simulink model "threebus"  (R2024a)
settings: Solver=VariableStepAuto  StartTime=0.0  StopTime=10.0  RelTol=1e-3
libraries: spsThreePhaseVIMeasurementLib x6, spsThreePhaseSeriesRLCBranchLib x3, spsLoadFlowBusLib x3, spsThreePhaseParallelRLCLoadLib x2, spsThreePhaseBreakerLib x1, spsThreePhaseSourceLib x1, sps_lib x1
settings Model: Creator=Vaibhav Chaudhary  LastModifiedBy=Vaibhav Chaudhary

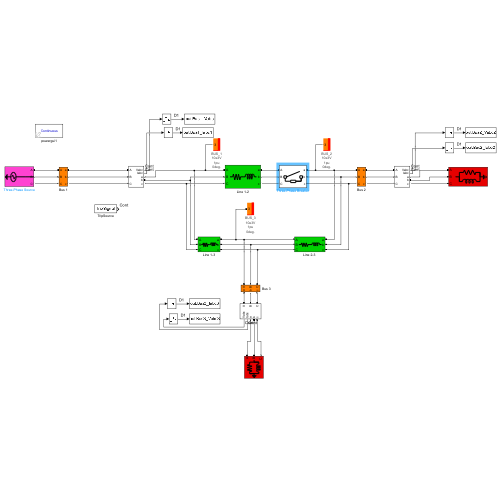
[thumbnail: Simulink's stored preview of the top-level diagram]
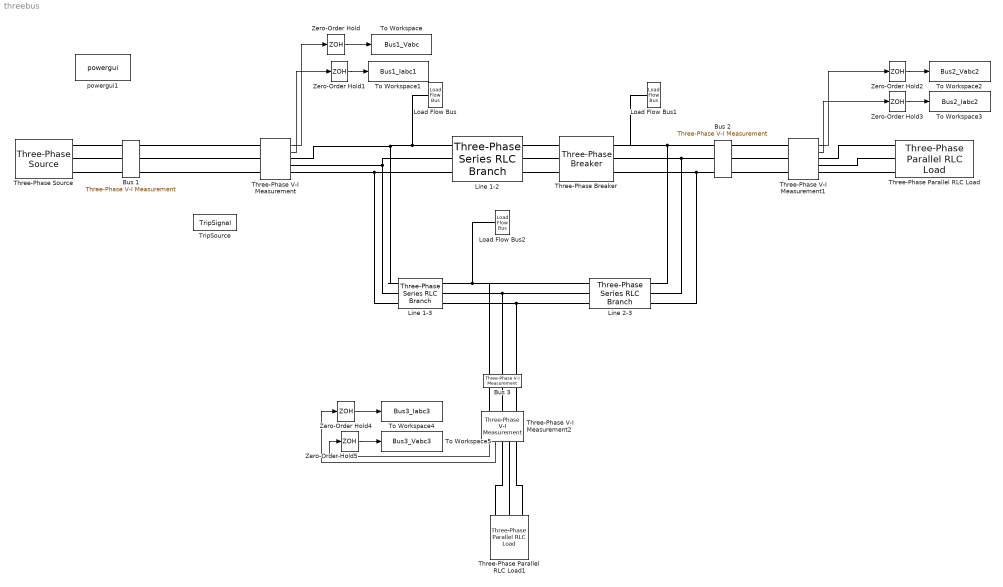
== system threebus ==
  Bus 1 : spsThreePhaseVIMeasurementLib/Three-Phase V-I Measurement  VoltageMeasurement=no  SetLabelV=off  LabelV=Vabc  Vpu=off  VpuLL=off  CurrentMeasurement=no  SetLabelI=off  LabelI=Iabc  Ipu=off  Pbase=100e6  Vbase=500e3  OutputType=Complex  PhasorSimulation=off  PSBequivalent=0
  Bus 2 : spsThreePhaseVIMeasurementLib/Three-Phase V-I Measurement  VoltageMeasurement=no  SetLabelV=off  LabelV=Vabc  Vpu=off  VpuLL=off  CurrentMeasurement=no  SetLabelI=off  LabelI=Iabc  Ipu=off  Pbase=100e6  Vbase=500e3  OutputType=Complex  PhasorSimulation=off  PSBequivalent=0
  Bus 3 : spsThreePhaseVIMeasurementLib/Three-Phase V-I Measurement  VoltageMeasurement=no  SetLabelV=off  LabelV=Vabc  Vpu=off  VpuLL=off  CurrentMeasurement=no  SetLabelI=off  LabelI=Iabc  Ipu=off  Pbase=100e6  Vbase=500e3  OutputType=Complex  PhasorSimulation=off  PSBequivalent=0
  Line 1-2 : spsThreePhaseSeriesRLCBranchLib/Three-Phase Series RLC Branch  LConnTagsString=A|B|C  RConnTagsString=A|B|C  BranchType=RL  Resistance=0.02  Inductance=106.1e-6  Capacitance=1e-6  Measurements=None
  Line 1-3 : spsThreePhaseSeriesRLCBranchLib/Three-Phase Series RLC Branch  LConnTagsString=A|B|C  RConnTagsString=A|B|C  BranchType=RL  Resistance=0.01  Inductance=79.577e-6  Capacitance=1e-6  Measurements=None
  "Line 2-3 " : spsThreePhaseSeriesRLCBranchLib/Three-Phase Series RLC Branch  LConnTagsString=A|B|C  RConnTagsString=A|B|C  BranchType=RL  Resistance=0.01  Inductance=66.31e-6  Capacitance=1e-6  Measurements=None
  Load Flow Bus : spsLoadFlowBusLib/Load Flow Bus  LConnTagsString=a  Phases=single  Connectors=on one side  ID=BUS_1  Vbase=10e3  Vref=1.05  Vangle=0  VLF=1  VLFb=1  VLFc=1  angleLF=0  angleLFb=0  angleLFc=0
  Load Flow Bus1 : spsLoadFlowBusLib/Load Flow Bus  LConnTagsString=a  Phases=single  Connectors=on one side  ID=BUS_2  Vbase=10e3  Vref=1.05  Vangle=0  VLF=1  VLFb=1  VLFc=1  angleLF=0  angleLFb=0  angleLFc=0
  Load Flow Bus2 : spsLoadFlowBusLib/Load Flow Bus  LConnTagsString=a  Phases=single  Connectors=on one side  ID=BUS_3  Vbase=10e3  Vref=1.05  Vangle=0  VLF=1  VLFb=1  VLFc=1  angleLF=0  angleLFb=0  angleLFc=0
  Three-Phase Parallel RLC Load : spsThreePhaseParallelRLCLoadLib/Three-Phase Parallel RLC Load  LConnTagsString=A|B|C  Configuration=Y (grounded)  NominalVoltage=1000  Vabc=[1e3 1e3 1e3]  Vabcp=[1e3 1e3 1e3]  NominalFrequency=60  UnbalancedPower=off  ActivePower=256.6e6  InductivePower=110.2e6  CapacitivePower=0  Pabc=[10e3 9e3 11e3]  QLabc=[100 90 110]  QCabc=[100 90 110]  Pabcp=[10e3 9e3 11e3]  QLabcp=[100 90 110]  QCabcp=[100 90 110]  Measurements=None  LoadType=constant PQ
  Three-Phase Parallel RLC Load1 : spsThreePhaseParallelRLCLoadLib/Three-Phase Parallel RLC Load  LConnTagsString=A|B|C  Configuration=Y (grounded)  NominalVoltage=1000  Vabc=[1e3 1e3 1e3]  Vabcp=[1e3 1e3 1e3]  NominalFrequency=60  UnbalancedPower=off  ActivePower=138.6e6  InductivePower=45.2e6  CapacitivePower=0  Pabc=[10e3 9e3 11e3]  QLabc=[100 90 110]  QCabc=[100 90 110]  Pabcp=[10e3 9e3 11e3]  QLabcp=[100 90 110]  QCabcp=[100 90 110]  Measurements=None  LoadType=constant PQ
  Three-Phase V-I Measurement : spsThreePhaseVIMeasurementLib/Three-Phase V-I Measurement  VoltageMeasurement=phase-to-ground  SetLabelV=off  LabelV=Vabc  Vpu=off  VpuLL=off  CurrentMeasurement=yes  SetLabelI=off  LabelI=Iabc  Ipu=off  Pbase=100e6  Vbase=500e3  OutputType=Complex  PhasorSimulation=off  PSBequivalent=0
  Three-Phase V-I Measurement1 : spsThreePhaseVIMeasurementLib/Three-Phase V-I Measurement  VoltageMeasurement=phase-to-ground  SetLabelV=off  LabelV=Vabc  Vpu=off  VpuLL=off  CurrentMeasurement=yes  SetLabelI=off  LabelI=Iabc  Ipu=off  Pbase=100e6  Vbase=500e3  OutputType=Complex  PhasorSimulation=off  PSBequivalent=0
  Three-Phase V-I Measurement2 : spsThreePhaseVIMeasurementLib/Three-Phase V-I Measurement  VoltageMeasurement=phase-to-ground  SetLabelV=off  LabelV=Vabc  Vpu=off  VpuLL=off  CurrentMeasurement=yes  SetLabelI=off  LabelI=Iabc  Ipu=off  Pbase=100e6  Vbase=500e3  OutputType=Complex  PhasorSimulation=off  PSBequivalent=0
  Three-Phase Breaker : spsThreePhaseBreakerLib/Three-Phase Breaker  InitialState=open  SwitchA=on  SwitchB=on  SwitchC=on  SwitchTimes="[1/60  5/60]"  External=off  BreakerResistance=0.01  SnubberResistance=1e6  SnubberCapacitance=inf  Measurements=None
  Three-Phase Source : spsThreePhaseSourceLib/Three-Phase Source  InternalConnection=Yg  VoltagePhases=off  Voltage=25e3  PhaseAngle=0  Voltage_phases=[25e3 25e3 25e3]/sqrt(3)  PhaseAngles_phases=[0 -120 +120]  Frequency=60  NonIdealSource=on  SpecifyImpedance=off  Resistance=0  Inductance=0  ShortCircuitLevel=100e6  BaseVoltage=25e3  XRratio=7  BusType=swing  Pref=10e3  Qref=0  Prefabc=[10e3, 10e3, 10e3]  Qrefabc=[0, 0, 0]  Qmin=-inf  Qmax=inf
  To Workspace : ToWorkspace  VariableName=Bus1_Vabc  SampleTime=-1
  To Workspace1 : ToWorkspace  VariableName=Bus1_Iabc1  SampleTime=-1
  To Workspace2 : ToWorkspace  VariableName=Bus2_Vabc2  SampleTime=-1
  To Workspace3 : ToWorkspace  VariableName=Bus2_Iabc2  SampleTime=-1
  To Workspace4 : ToWorkspace  VariableName=Bus3_Iabc3  SampleTime=-1
  To Workspace5 : ToWorkspace  VariableName=Bus3_Vabc3  SampleTime=-1
  TripSource : FromWorkspace  VariableName=TripSignal
  Zero-Order Hold{,1..5} (6 alike) : ZeroOrderHold  SampleTime=0.1
  powergui1 : sps_lib/powergui  Priority=1  SimulationMode=Continuous  SampleTime=50e-6  frequency=60  Iterations=50  frequencyindice=60  Pbase=100e6  ErrMax=1e-4  UnitsV=kV  UnitsW=MW  buscounter=0  FunctionMessages=off  echomessages=off  EnableUseOfTLC=off  CurrentSourceSwitches=off  DisableSnubberDevices=off  DisableRonSwitches=off  DisableVfSwitches=off  DisplayEquations=off  AutomaticDiscreteSolvers=off  SolverType=Tustin/Backward Euler (TBE)  Interpol=off  ExternalGateDelay=off  methode=off  Ts=100  x0status=blocks  SPID=on  SwTol=0  HookPort=off  NonlinearTolerance=1e-4  nMaxIteration=100  ContinueOnMaxIteration=off  RestoreLinks=warning  ResistiveCurrentMeasurement=off  Frange=[0:2:500]  Ylog=off  Xlog=on  ShowGrid=off  save=off  variable=ZData  structure=0  ZoomFFT=off  StartTime=0.0  cycles=1  DisplayStyle=1  fundamental=60  FreqAxis=off  MaxFrequency=1000  frequencyindicesteady=1  RmsSteady=1  display=off
  wires:
  Zero-Order Hold/1 -> To Workspace/1
  Three-Phase V-I Measurement/1 -> Zero-Order Hold/1
  Zero-Order Hold1/1 -> To Workspace1/1
  Three-Phase V-I Measurement/2 -> Zero-Order Hold1/1
  Zero-Order Hold2/1 -> To Workspace2/1
  Three-Phase V-I Measurement1/1 -> Zero-Order Hold2/1
  Zero-Order Hold3/1 -> To Workspace3/1
  Three-Phase V-I Measurement1/2 -> Zero-Order Hold3/1
  Zero-Order Hold4/1 -> To Workspace4/1
  Three-Phase V-I Measurement2/2 -> Zero-Order Hold4/1
  Zero-Order Hold5/1 -> To Workspace5/1
  Three-Phase V-I Measurement2/1 -> Zero-Order Hold5/1
  connections:
  Three-Phase Source/RConn1 -- Bus 1/LConn1
  Three-Phase Source/RConn2 -- Bus 1/LConn2
  Three-Phase Source/RConn3 -- Bus 1/LConn3
  Line 1-3/LConn1 -- Three-Phase V-I Measurement/RConn1 -- Line 1-2/LConn1 -- Load Flow Bus/LConn1
  Line 1-3/LConn2 -- Line 1-2/LConn2 -- Three-Phase V-I Measurement/RConn2
  Line 1-3/LConn3 -- Line 1-2/LConn3 -- Three-Phase V-I Measurement/RConn3
  Bus 2/LConn1 -- Three-Phase Breaker/RConn1 -- Load Flow Bus1/LConn1 -- "Line 2-3 "/RConn1
  "Line 2-3 "/RConn2 -- Bus 2/LConn2 -- Three-Phase Breaker/RConn2
  "Line 2-3 "/RConn3 -- Bus 2/LConn3 -- Three-Phase Breaker/RConn3
  "Line 2-3 "/LConn3 -- Bus 3/LConn3 -- Line 1-3/RConn3
  "Line 2-3 "/LConn2 -- Line 1-3/RConn2 -- Bus 3/LConn2
  Line 1-3/RConn1 -- Bus 3/LConn1 -- "Line 2-3 "/LConn1 -- Load Flow Bus2/LConn1
  Bus 1/RConn3 -- Three-Phase V-I Measurement/LConn3
  Bus 1/RConn2 -- Three-Phase V-I Measurement/LConn2
  Bus 1/RConn1 -- Three-Phase V-I Measurement/LConn1
  Three-Phase V-I Measurement1/LConn3 -- Bus 2/RConn3
  Three-Phase V-I Measurement1/LConn2 -- Bus 2/RConn2
  Three-Phase V-I Measurement1/LConn1 -- Bus 2/RConn1
  Three-Phase V-I Measurement1/RConn3 -- Three-Phase Parallel RLC Load/LConn3
  Three-Phase V-I Measurement1/RConn2 -- Three-Phase Parallel RLC Load/LConn2
  Three-Phase V-I Measurement1/RConn1 -- Three-Phase Parallel RLC Load/LConn1
  Three-Phase V-I Measurement2/RConn1 -- Three-Phase Parallel RLC Load1/LConn1
  Three-Phase V-I Measurement2/RConn2 -- Three-Phase Parallel RLC Load1/LConn2
  Three-Phase V-I Measurement2/RConn3 -- Three-Phase Parallel RLC Load1/LConn3
  Bus 3/RConn3 -- Three-Phase V-I Measurement2/LConn3
  Bus 3/RConn2 -- Three-Phase V-I Measurement2/LConn2
  Bus 3/RConn1 -- Three-Phase V-I Measurement2/LConn1
  Three-Phase Breaker/LConn1 -- Line 1-2/RConn1
  Three-Phase Breaker/LConn2 -- Line 1-2/RConn2
  Three-Phase Breaker/LConn3 -- Line 1-2/RConn3
